simulink model "ReadyToGoControlCircuit"  (R2016a)
settings: Solver=VariableStepAuto  StartTime=0.0  StopTime=10.0  RelTol=1e-3
settings Model: Creator=METZLER  LastModifiedBy=chris.barlow
settings DataIOCC: LimitDataPoints=on
settings DebuggingCC: AllowSymbolicDim=off
settings ModelReferenceCC: PropagateSignalLabelsOutOfModel=off
settings GRTTargetCC: GeneratePreprocessorConditionals=Use local settings

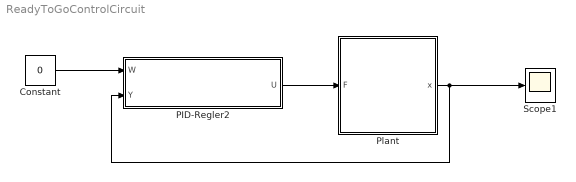
== system ReadyToGoControlCircuit ==
  Constant : Constant  Value=0
  PID-Regler2 : Subsystem  mask{cpc=0.5, cic=0, cdc=0, T=0.1}
      mask prompts: T "T  Time constant of real D-Part"
      mask help: A simple PID-Controller for the MOOC MSUS
      mask Display:
      | IconText='';
      | if ~strcmp(get_param(gcb,'cpc'),'0')
      |     IconText=strcat(IconText,'P');
      | end
      | if ~strcmp(get_param(gcb,'cic'),'0')
      |    IconText=strcat(IconText,'I');
      | end
      | if ~strcmp(get_param(gcb,'cdc'),'0')
      |     IconText=strcat(IconText,'D');
      | end
      | IconText=strcat(IconText,'-Controller')
      | plot(0,0)
      | plot(100,100)
      | text(25,50,IconText)
      | port_label ('output',1,'U')
      | port_label ('input',1,'W')
      | port_label ('input',2,'Y')
  Plant : Subsystem  mask{v0=0, X0=2, C=1, D=0, m=1}
      mask prompts: v0 "Initial Speed v0 [m/s]"; X0 "Initial Position x0 [m]"; C "Spring Constant C [N/m]"; D "Damper Constant D [Ns/m]"; m "Mass m [kg]"
      mask help:
      | A simple mass spring damper system to resemble
      | a simple control plantfor the MOOC MSUS
      mask Display:
      | plot(0,0)
      | plot(100,100)
      | 
      | plot([20 70],[80 80])
      | plot([30 40],[80 90])
      | plot([45 55],[80 90])
      | plot([60 70],[80 90])
      | 
      | patch([30 40 40 30],[55 55 60 60],[0 0 0 ])
      | plot([28 28],[63 50])
      | plot([42 42],[63 50])
      | plot([28 42],[50 50])
      | plot([35 35],[60 80])
      | plot([35 35],[50 30])
      | 
      | patch([10 80 80 10],[25 25 39 39],[0.9 0.8 0.3])
      | text(44,32,'m')
      | plot([10 80],[25 25])
      | plot([10 80],[39 39])
      | plot([10 10],[25 39])
      | plot([80 80],[25 39])
      | 
      | plot([60 60],[80 70])
      | plot([60 55],[70 68])
      | plot([55 65],[68 64])
      | plot([65 55],[64 60])
      | plot([55 65],[60 55])
      | plot([55 65],[51 55])
      | plot([55 60],[51 49])
      | plot([60 60],[49 39])
      | 
      | plot([45 45],[25 5])
      | 
      | patch([42 45 48],[10 5 10],[0  0 0])
      | 
      | text(50,15,'F, x')
      | text(70,60,'C')
      | text(20,60,'D')
      | 
      | port_label ('output',1,'x')
      | port_label ('input',1,'F')
  Scope1 : Scope
  wires:
  PID-Regler2/1(U) -> Plant/1(F)
  Plant/1(x) -> Scope1/1, PID-Regler2/2(Y)
  Constant/1 -> PID-Regler2/1(W)

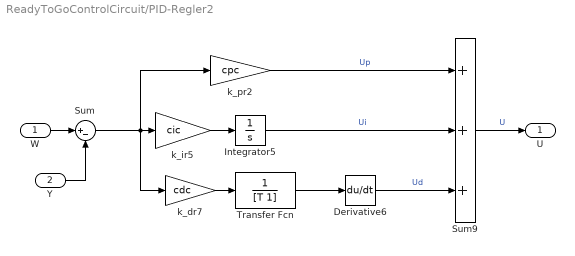
== system ReadyToGoControlCircuit/PID-Regler2 ==
  W : Inport
  Y : Inport  Port=2
  Derivative6 : Derivative
  Integrator5 : Integrator
  Sum : Sum  Inputs=|+-
  Sum9 : Sum  Inputs=+++
  Transfer Fcn : TransferFcn  Denominator=[T 1]
  k_dr7 : Gain  Gain=cdc
  k_ir5 : Gain  Gain=cic
  k_pr2 : Gain  Gain=cpc
  U : Outport
  wires:
  Y/1 -> Sum/2
  Sum9/1 -> U/1  "U"
  W/1 -> Sum/1
  Derivative6/1 -> Sum9/3  "Ud"
  k_pr2/1 -> Sum9/1  "Up"
  k_ir5/1 -> Integrator5/1
  Integrator5/1 -> Sum9/2  "Ui"
  Transfer Fcn/1 -> Derivative6/1
  k_dr7/1 -> Transfer Fcn/1
  Sum/1 -> k_ir5/1, k_pr2/1, k_dr7/1

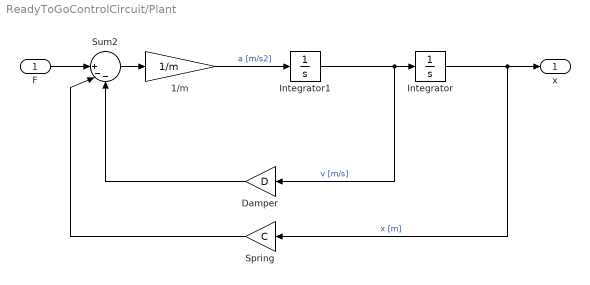
== system ReadyToGoControlCircuit/Plant ==
  F : Inport
  1/m : Gain  Gain=1/m
  Damper : Gain  Gain=D
  Integrator : Integrator  InitialCondition=X0
  Integrator1 : Integrator  InitialCondition=v0
  Spring : Gain  Gain=C
  Sum2 : Sum  Inputs=||+--
  x : Outport
  wires:
  Integrator/1 -> x/1, Spring/1  "x [m]"
  1/m/1 -> Integrator1/1  "a [m/s2]"
  Integrator1/1 -> Integrator/1, Damper/1  "v [m/s]"
  Sum2/1 -> 1/m/1
  Damper/1 -> Sum2/3
  Spring/1 -> Sum2/2
  F/1 -> Sum2/1
